simulink model "robot_action"  (R2014b)
settings: Solver=ode45  StartTime=0.0  StopTime=10  FixedStep=1e-4  RelTol=1e-3
values from neighbouring files (symbols this model uses):
  robot_floor_friction_coeff = 0.6    [robot_init.m]
  robot_floor_position_gain = -1e5    (= -100000)    [robot_init.m]
  robot_floor_speed_gain = -1e3    (= -1000)    [robot_init.m]
  robot_gravity = [0 0 -9.80665]    [robot_init.m]
undefined symbols (not defined in the file or in its folder): CM730_acc_center, CM730_acc_gain, CM730_gyro_center, CM730_gyro_gain, CM730_sample_time, FSR_max, FSR_no_load, FSR_sample_time, FSR_scale, MX28_inertia, MX28_Te, X, Y, Z
libraries: sm_lib x158, fl_lib x128, nesl_utility x77
(part 6 of 6)

== system robot_action/Right Leg/Floor model/Floor Model Front Right ==
  6-DOF Joint1 : sm_lib/Joints/6-DOF Joint  SenseConstraintForce=off  SenseConstraintForceX=off  SenseConstraintForceY=off  SenseConstraintForceZ=off  SenseConstraintTorque=off  SenseConstraintTorqueX=off  SenseConstraintTorqueY=off  SenseConstraintTorqueZ=off  SenseTotalForce=off  SenseTotalForceX=off  SenseTotalForceY=off  SenseTotalForceZ=off  SenseTotalTorque=off  SenseTotalTorqueX=off  SenseTotalTorqueY=off  SenseTotalTorqueZ=off  CompositeWrenchDir=FollowerOnBase  CompositeWrenchFrame=BaseFrame  PxEquilibriumPosition=0  PxEquilibriumPositionUnits=m  PxSpringStiffness=0  PxSpringStiffnessUnits=N/m  PxDampingCoefficient=0  PxDampingCoefficientUnits=N/(m/s)  PxTorqueActuationMode=InputTorque  PxMotionActuationMode=ComputedMotion  PxSensePosition=off  PxSenseVelocity=on  PxSenseAcceleration=off  PxSenseTorqueForce=off  PxPositionTargetValue=0  PxPositionTargetValueUnits=m  PxPositionTargetSpecify=off  PxPositionTargetPriority=High  PxVelocityTargetValue=0  PxVelocityTargetValueUnits=m/s  PxVelocityTargetSpecify=off  PxVelocityTargetPriority=High  PyEquilibriumPosition=0  PyEquilibriumPositionUnits=m  PySpringStiffness=0  PySpringStiffnessUnits=N/m  PyDampingCoefficient=0  PyDampingCoefficientUnits=N/(m/s)  PyTorqueActuationMode=InputTorque  PyMotionActuationMode=ComputedMotion  PySensePosition=off  PySenseVelocity=on  PySenseAcceleration=off  PySenseTorqueForce=off  PyPositionTargetValue=0  PyPositionTargetValueUnits=m  PyPositionTargetSpecify=off  PyPositionTargetPriority=High  PyVelocityTargetValue=0  PyVelocityTargetValueUnits=m/s  PyVelocityTargetSpecify=off  PyVelocityTargetPriority=High  PzEquilibriumPosition=0  PzEquilibriumPositionUnits=m  PzSpringStiffness=0  PzSpringStiffnessUnits=N/m  PzDampingCoefficient=0  PzDampingCoefficientUnits=N/(m/s)  PzTorqueActuationMode=InputTorque  PzMotionActuationMode=ComputedMotion  PzSensePosition=on  PzSenseVelocity=on  PzSenseAcceleration=off  PzSenseTorqueForce=off  PzPositionTargetValue=0  PzPositionTargetValueUnits=m  PzPositionTargetSpecify=off  PzPositionTargetPriority=High  PzVelocityTargetValue=0  PzVelocityTargetValueUnits=m/s  PzVelocityTargetSpecify=off  PzVelocityTargetPriority=High  SphDefPosRotationMethod=None  SphDefPosRotationAngleUnits=deg  SphDefPosRotationStandardAxis=+Z  SphDefPosRotationAngle=0.0  SphDefPosRotationArbitraryAxis=[0 0 1]  SphDefPosFollAlignAxisA=+X  SphDefPosBaseAlignAxisA=+Y  SphDefPosFollAlignAxisB=+Y  SphDefPosBaseAlignAxisB=+Z  SphDefPosRotationMatrix=[1 0 0; 0 1 0; 0 0 1]  SphEqPosRotationMethod=None  SphEqPosRotationAngleUnits=deg  SphEqPosRotationStandardAxis=+Z  SphEqPosRotationAngle=0.0  SphEqPosRotationArbitraryAxis=[0 0 1]  SphEqPosFollAlignAxisA=+X  SphEqPosBaseAlignAxisA=+Y  SphEqPosFollAlignAxisB=+Y  SphEqPosBaseAlignAxisB=+Z  SphEqPosRotationMatrix=[1 0 0; 0 1 0; 0 0 1]  SphSpringStiffness=0  SphSpringStiffnessUnits=N*m/deg  SphDampingCoefficient=0  SphDampingCoefficientUnits=N*m/(deg/s)  SphActuateTorqueX=off  SphActuateTorqueY=off  SphActuateTorqueZ=off  SphActuateTorque=off  SphTorqueActuationMode=NoTorque  SphMotionActuationMode=ComputedMotion  SphActuationFrame=BaseFrame  SphSensePosition=off  SphSenseVelocityX=off  SphSenseVelocityY=off  SphSenseVelocityZ=off  SphSenseVelocity=off  SphSenseAccelerationX=off  SphSenseAccelerationY=off  SphSenseAccelerationZ=off  SphSenseAcceleration=off  SphSenseTorqueX=off  SphSenseTorqueY=off  SphSenseTorqueZ=off  SphSenseTorqueForce=off  SphSensingFrame=BaseFrame  SphPositionTargetRotationMethod=None  SphPositionTargetRotationAngleUnits=deg  SphPositionTargetRotationStandardAxis=+Z  SphPositionTargetRotationAngle=0.0  SphPositionTargetRotationArbitraryAxis=[0 0 1]  SphPositionTargetFollAlignAxisA=+X  SphPositionTargetBaseAlignAxisA=+Y  SphPositionTargetFollAlignAxisB=+Y  SphPositionTargetBaseAlignAxisB=+Z  SphPositionTargetRotationMatrix=[1 0 0; 0 1 0; 0 0 1]  SphPositionTargetSpecify=off  SphPositionTargetPriority=High  SphVelocityTargetValue=[0 0 0]  SphVelocityTargetValueUnits=deg/s  SphVelocityTargetSpecify=off  SphVelocityTargetPriority=High  SphVelocityTargetInFollowerFrame=on  BlockFunction=simmechanics.library.joints.sixdof_joint
  Friction coeff : fl_lib/Physical Signals/Functions/PS Gain  gain=robot_floor_friction_coeff
  No friction : fl_lib/Physical Signals/Sources/PS Constant  constant=0
  PS Abs : fl_lib/Physical Signals/Nonlinear Operators/PS Abs
  PS-Simulink Converter : nesl_utility/PS-Simulink Converter  PhysicalDomain=network_engine_domain  SubClassName=ps_output  LeftPortType=input  RightPortType=output  PseudoPeriodic=off  Frequencies=[]  Unit=N  AffineConversion=off
  Saturation : Saturate  UpperLimit=+inf  LowerLimit=0
  Unary minus : fl_lib/Physical Signals/Functions/PS Gain  gain=-1
  X Lower Bound : fl_lib/Physical Signals/Nonlinear Operators/PS Max
  X Speed Gain : fl_lib/Physical Signals/Functions/PS Gain  gain=robot_floor_speed_gain
  X Switch : fl_lib/Physical Signals/Nonlinear Operators/PS Switch  Threshold=0
  X Upper Bound : fl_lib/Physical Signals/Nonlinear Operators/PS Min
  Y Lower Bound : fl_lib/Physical Signals/Nonlinear Operators/PS Max
  Y Speed Gain : fl_lib/Physical Signals/Functions/PS Gain  gain=robot_floor_speed_gain
  Y Switch : fl_lib/Physical Signals/Nonlinear Operators/PS Switch  Threshold=0
  Y Upper Bound : fl_lib/Physical Signals/Nonlinear Operators/PS Min
  Z Add : fl_lib/Physical Signals/Functions/PS Add
  Z Position Gain : fl_lib/Physical Signals/Functions/PS Gain  gain=robot_floor_position_gain
  Z Speed Gain : fl_lib/Physical Signals/Functions/PS Gain  gain=robot_floor_speed_gain
  Z Switch : fl_lib/Physical Signals/Nonlinear Operators/PS Switch  Threshold=0
  Contact : PMIOPort  Port=1  Side=Left
  Floor : PMIOPort  Port=2  Side=Right
  Z force : Outport
  wires:
  PS-Simulink Converter/1 -> Saturation/1
  Saturation/1 -> Z force/1
  connections:
  Floor/RConn1 -- 6-DOF Joint1/LConn1
  6-DOF Joint1/RConn1 -- Contact/RConn1
  No friction/RConn1 -- Y Switch/LConn1 -- Z Switch/LConn1 -- X Switch/LConn1
  Z Position Gain/RConn1 -- Z Add/LConn1
  Z Switch/LConn3 -- Z Add/RConn1 -- Friction coeff/LConn1 -- PS-Simulink Converter/LConn1
  Z Speed Gain/RConn1 -- Z Add/LConn2
  6-DOF Joint1/RConn5 -- Z Speed Gain/LConn1
  6-DOF Joint1/LConn4 -- Z Switch/RConn1
  Z Switch/LConn2 -- Z Position Gain/LConn1 -- 6-DOF Joint1/RConn4 -- X Switch/LConn2 -- Y Switch/LConn2
  Y Switch/RConn1 -- 6-DOF Joint1/LConn3
  Y Speed Gain/LConn1 -- 6-DOF Joint1/RConn3
  PS Abs/LConn1 -- Friction coeff/RConn1
  PS Abs/RConn1 -- Unary minus/LConn1 -- X Upper Bound/LConn2 -- Y Upper Bound/LConn2
  Y Upper Bound/RConn1 -- Y Lower Bound/LConn1
  Y Lower Bound/LConn2 -- Unary minus/RConn1 -- X Lower Bound/LConn2
  Y Lower Bound/RConn1 -- Y Switch/LConn3
  Y Upper Bound/LConn1 -- Y Speed Gain/RConn1
  X Speed Gain/LConn1 -- 6-DOF Joint1/RConn2
  X Upper Bound/LConn1 -- X Speed Gain/RConn1
  X Lower Bound/LConn1 -- X Upper Bound/RConn1
  X Switch/LConn3 -- X Lower Bound/RConn1
  X Switch/RConn1 -- 6-DOF Joint1/LConn2

== stateflow chart robot_action/Action FSM ==
  settings: updateMethod=DISCRETE  sampleTime=0.008
  state Action_Init_State
    entry: running = true;
    entry: Apply_Slopes();
    entry: step_index = uint16(1);
  state Initialization_State
    entry: running = false;
    exit: action_index = start_action_index;
  state Action_External_Next_Action
    entry: action_index = next_action_index;
  state Action_Pause
    entry: delay = int16(robot_actions.steppause(action_index,step_index));
    during: delay = delay - 1;
  state Action_Move
    entry: Apply_Position_Speed();
    entry: delay = int16(robot_actions.steptime(action_index,step_index));
    during: delay = delay - 1;
  state Action_Internal_Next_Action
    entry: action_index = int16(robot_actions.next(action_index))+1;
  state Action_Next_Step
    entry: step_index = step_index+1;
  (default) -> Initialization_State
  Action_External_Next_Action -> Initialization_State [order 2] : [action_index == 0]
  Initialization_State -> Action_Init_State : [start_action_index > 0]
  Action_External_Next_Action -> Action_Init_State [order 1] : [action_index > 0]
  Action_Internal_Next_Action -> Action_Init_State [order 2] : [action_index > 1]
  Action_Init_State -> Action_Pause : [1]
  Action_Internal_Next_Action -> Action_External_Next_Action [order 1] : [action_index == 1]
  Action_Next_Step -> Action_Pause [order 1] : [step_index <= robot_actions.stepnum(action_index)]
  Action_Pause -> Action_Move : [delay <= 0]
  Action_Move -> Action_Next_Step : [delay <= 0]
  Action_Next_Step -> Action_Internal_Next_Action [order 2] : [step_index > robot_actions.stepnum(action_index)]
  data: MX28_ID1 data_store_memory; MX28_ID2 data_store_memory; MX28_ID3 data_store_memory; MX28_ID4 data_store_memory; MX28_ID5 data_store_memory; MX28_ID6 data_store_memory; MX28_ID7 data_store_memory; MX28_ID8 data_store_memory; MX28_ID9 data_store_memory; MX28_ID10 data_store_memory; MX28_ID11 data_store_memory; MX28_ID12 data_store_memory; MX28_ID13 data_store_memory; MX28_ID14 data_store_memory; MX28_ID15 data_store_memory; MX28_ID16 data_store_memory; MX28_ID17 data_store_memory; MX28_ID18 data_store_memory; MX28_ID19 data_store_memory; MX28_ID20 data_store_memory; CM730_ID200 data_store_memory; FSR_ID111 data_store_memory; FSR_ID112 data_store_memory; delay local int16 =0; start_action_index input int16; action_index local int16; step_index local uint16; robot_actions data_store_memory size=[1 256]; running output boolean; next_action_index input int16
  function Apply_Slopes:
    | function Apply_Slopes
    |     MX28_ID1.P_gain  = calc_slope(robot_actions.slope(action_index,2));
    |     MX28_ID2.P_gain  = calc_slope(robot_actions.slope(action_index,3));
    |     MX28_ID3.P_gain  = calc_slope(robot_actions.slope(action_index,4));
    |     MX28_ID4.P_gain  = calc_slope(robot_actions.slope(action_index,5));
    |     MX28_ID5.P_gain  = calc_slope(robot_actions.slope(action_index,6));
    |     MX28_ID6.P_gain  = calc_slope(robot_actions.slope(action_index,7));
    |     MX28_ID7.P_gain  = calc_slope(robot_actions.slope(action_index,8));
    |     MX28_ID8.P_gain  = calc_slope(robot_actions.slope(action_index,9));
    |     MX28_ID9.P_gain  = calc_slope(robot_actions.slope(action_index,10));
    |     MX28_ID10.P_gain = calc_slope(robot_actions.slope(action_index,11));
    |     MX28_ID11.P_gain = calc_slope(robot_actions.slope(action_index,12));
    |     MX28_ID12.P_gain = calc_slope(robot_actions.slope(action_index,13));
    |     MX28_ID13.P_gain = calc_slope(robot_actions.slope(action_index,14));
    |     MX28_ID14.P_gain = calc_slope(robot_actions.slope(action_index,15));
    |     MX28_ID15.P_gain = calc_slope(robot_actions.slope(action_index,16));
    |     MX28_ID16.P_gain = calc_slope(robot_actions.slope(action_index,17));
    |     MX28_ID17.P_gain = calc_slope(robot_actions.slope(action_index,18));
    |     MX28_ID18.P_gain = calc_slope(robot_actions.slope(action_index,19));
    |     MX28_ID19.P_gain = calc_slope(robot_actions.slope(action_index,20));
    |     MX28_ID20.P_gain = calc_slope(robot_actions.slope(action_index,21));
    | end
    | 
    | function s = calc_slope(raw)
    |     s = uint8(floor(256/2^floor(double(raw)/16))*4);
    | end
  function Apply_Position_Speed:
    | function Apply_Position_Speed
    | 
    | speed_ratio = 1024 / (double(robot_actions.steptime(action_index,step_index)) * 8) / 8;
    | 
    | MX28_ID1.moving_speed = int16(double(abs(MX28_ID1.goal_position - robot_actions.stepposition(action_index,step_index,2))) * speed_ratio);
    | MX28_ID1.goal_position = robot_actions.stepposition(action_index,step_index,2);
    | 
    | MX28_ID2.moving_speed = int16(double(abs(MX28_ID2.goal_position - robot_actions.stepposition(action_index,step_index,3))) * speed_ratio);
    | MX28_ID2.goal_position = robot_actions.stepposition(action_index,step_index,3);
    | 
    | MX28_ID3.moving_speed = int16(double(abs(MX28_ID3.goal_position - robot_actions.stepposition(action_index,step_index,4))) * speed_ratio);
    | MX28_ID3.goal_position = robot_actions.stepposition(action_index,step_index,4);
    | 
    | MX28_ID4.moving_speed = int16(double(abs(MX28_ID4.goal_position - robot_actions.stepposition(action_index,step_index,5))) * speed_ratio);
    | MX28_ID4.goal_position = robot_actions.stepposition(action_index,step_index,5);
    | 
    | MX28_ID5.moving_speed = int16(double(abs(MX28_ID5.goal_position - robot_actions.stepposition(action_index,step_index,6))) * speed_ratio);
    | MX28_ID5.goal_position = robot_actions.stepposition(action_index,step_index,6);
    | 
    | MX28_ID6.moving_speed = int16(double(abs(MX28_ID6.goal_position - robot_actions.stepposition(action_index,step_index,7))) * speed_ratio);
    | MX28_ID6.goal_position = robot_actions.stepposition(action_index,step_index,7);
    | 
    | MX28_ID7.moving_speed = int16(double(abs(MX28_ID7.goal_position - robot_actions.stepposition(action_index,step_index,8))) * speed_ratio);
    | MX28_ID7.goal_position = robot_actions.stepposition(action_index,step_index,8);
    | 
    | MX28_ID8.moving_speed = int16(double(abs(MX28_ID8.goal_position - robot_actions.stepposition(action_index,step_index,9))) * speed_ratio);
    | MX28_ID8.goal_position = robot_actions.stepposition(action_index,step_index,9);
    | 
    | MX28_ID9.moving_speed = int16(double(abs(MX28_ID9.goal_position - robot_actions.stepposition(action_index,step_index,10))) * speed_ratio);
    | MX28_ID9.goal_position = robot_actions.stepposition(action_index,step_index,10);
    | 
    | MX28_ID10.moving_speed = int16(double(abs(MX28_ID10.goal_position - robot_actions.stepposition(action_index,step_index,11))) * speed_ratio);
    | MX28_ID10.goal_position = robot_actions.stepposition(action_index,step_index,11);
    | 
    | MX28_ID11.moving_speed = int16(double(abs(MX28_ID11.goal_position - robot_actions.stepposition(action_index,step_index,12))) * speed_ratio);
    | MX28_ID11.goal_position = robot_actions.stepposition(action_index,step_index,12);
    | 
    | MX28_ID12.moving_speed = int16(double(abs(MX28_ID12.goal_position - robot_actions.stepposition(action_index,step_index,13))) * speed_ratio);
    | MX28_ID12.goal_position = robot_actions.stepposition(action_index,step_index,13);
    | 
    | MX28_ID13.moving_speed = int16(double(abs(MX28_ID13.goal_position - robot_actions.stepposition(action_index,step_index,14))) * speed_ratio);
    | MX28_ID13.goal_position = robot_actions.stepposition(action_index,step_index,14);
    | 
    | MX28_ID14.moving_speed = int16(double(abs(MX28_ID14.goal_position - robot_actions.stepposition(action_index,step_index,15))) * speed_ratio);
    | MX28_ID14.goal_position = robot_actions.stepposition(action_index,step_index,15);
    | 
    | MX28_ID15.moving_speed = int16(double(abs(MX28_ID15.goal_position - robot_actions.stepposition(action_index,step_index,16))) * speed_ratio);
    | MX28_ID15.goal_position = robot_actions.stepposition(action_index,step_index,16);
    | 
    | MX28_ID16.moving_speed = int16(double(abs(MX28_ID16.goal_position - robot_actions.stepposition(action_index,step_index,17))) * speed_ratio);
    | MX28_ID16.goal_position = robot_actions.stepposition(action_index,step_index,17);
    | 
    | MX28_ID17.moving_speed = int16(double(abs(MX28_ID17.goal_position - robot_actions.stepposition(action_index,step_index,18))) * speed_ratio);
    | MX28_ID17.goal_position = robot_actions.stepposition(action_index,step_index,18);
    | 
    | MX28_ID18.moving_speed = int16(double(abs(MX28_ID18.goal_position - robot_actions.stepposition(action_index,step_index,19))) * speed_ratio);
    | MX28_ID18.goal_position = robot_actions.stepposition(action_index,step_index,19);
    | 
    | MX28_ID19.moving_speed = int16(double(abs(MX28_ID19.goal_position - robot_actions.stepposition(action_index,step_index,20))) * speed_ratio);
    | MX28_ID19.goal_position = robot_actions.stepposition(action_index,step_index,20);
    | 
    | MX28_ID20.moving_speed = int16(double(abs(MX28_ID20.goal_position - robot_actions.stepposition(action_index,step_index,21))) * speed_ratio);
    | MX28_ID20.goal_position = robot_actions.stepposition(action_index,step_index,21);
